simulink model "graduteWork"  (R2019b)
settings: Solver=VariableStepAuto  StartTime=0.0  StopTime=30  RelTol=1e-6  AbsTol=1e-6
values from neighbouring files (symbols this model uses):
  G_0 = db2mag(94)    [apll_attr.m]    (also in apll_const.m = db2mag(90.8); test.m = db2mag(87.3))
  K = 3    [constants.m]    (also in main.m; test.m)
  omega_0 = 0    [apll_attr.m]    (also in apll_const.m; test.m)
  T_b = 2    [constants.m]    (also in main.m)
  tau_p1 = 1.65*1e-3    (= 0.00165)    [apll_attr.m]    (also in apll_attr_nondim_1.m; apll_attr_nondim_2.m; apll_attr_nondim_3.m; apll_const.m)
  tau_p2 = 1.65*1e-3    (= 0.00165)    [apll_attr.m]    (also in apll_attr_nondim_1.m; apll_attr_nondim_2.m; apll_attr_nondim_3.m; apll_const.m)
  tau_z1 = 165*1e-6    (= 0.000165)    [apll_attr.m]    (also in apll_attr_nondim_1.m; apll_attr_nondim_2.m; apll_attr_nondim_3.m; apll_const.m)
  tau_z2 = 165*1e-6    (= 0.000165)    [apll_attr.m]    (also in apll_attr_nondim_1.m; apll_attr_nondim_2.m; apll_attr_nondim_3.m; apll_const.m)
libraries: simulink x3, commrandsrc3 x1, commutil2 x1
settings Model: Creator=Elena  LastModifiedBy=Elena

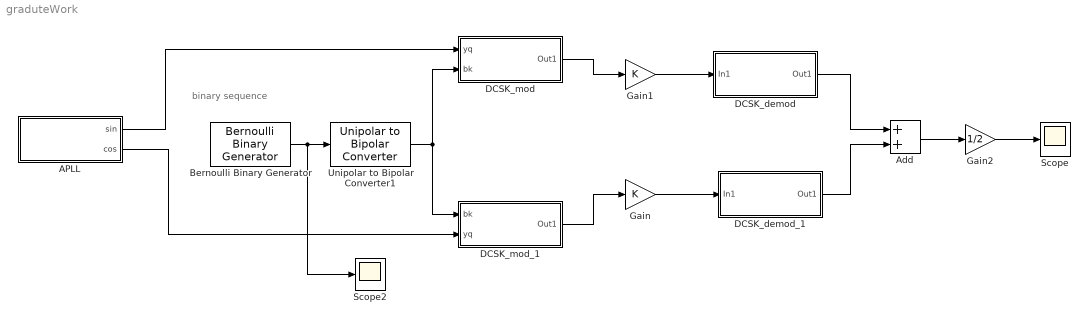
== system graduteWork ==
  note: binary sequence
  "APLL " : Subsystem
  Add : Sum
  Bernoulli Binary Generator : commrandsrc3/Bernoulli Binary Generator  ProbabilityOfZero=0.5  SeedSource=Auto  Seed=0  SampleTime=T_b  SamplesPerFrame=1  OutputDataType=double  SimulateUsing=Interpreted execution
      settings: SourceProductName=Communications Toolbox
  "DCSK_demod " : Subsystem
  "DCSK_demod_1 " : Subsystem
  DCSK_mod : Subsystem
  DCSK_mod_1 : Subsystem
  Gain : Gain  Gain=K
  Gain1 : Gain  Gain=K
  Gain2 : Gain  Gain=1/2
  Scope : Scope
  Scope2 : Scope
  Unipolar to Bipolar Converter1 : commutil2/Unipolar to Bipolar Converter  M=2  polarity=Positive  dataType=Inherit via internal rule
      settings: SourceProductName=Communications Toolbox
  wires:
  "APLL "/1(sin) -> DCSK_mod/1(yq)
  DCSK_mod/1(Out1) -> Gain1/1
  DCSK_mod_1/1(Out1) -> Gain/1
  Add/1 -> Gain2/1
  Unipolar to Bipolar Converter1/1 -> DCSK_mod/2(bk), DCSK_mod_1/1(bk)
  Bernoulli Binary Generator/1 -> Unipolar to Bipolar Converter1/1, Scope2/1
  "APLL "/2(cos) -> DCSK_mod_1/2(yq)
  "DCSK_demod_1 "/1(Out1) -> Add/2
  "DCSK_demod "/1(Out1) -> Add/1
  Gain1/1 -> "DCSK_demod "/1(In1)
  Gain/1 -> "DCSK_demod_1 "/1(In1)
  Gain2/1 -> Scope/1

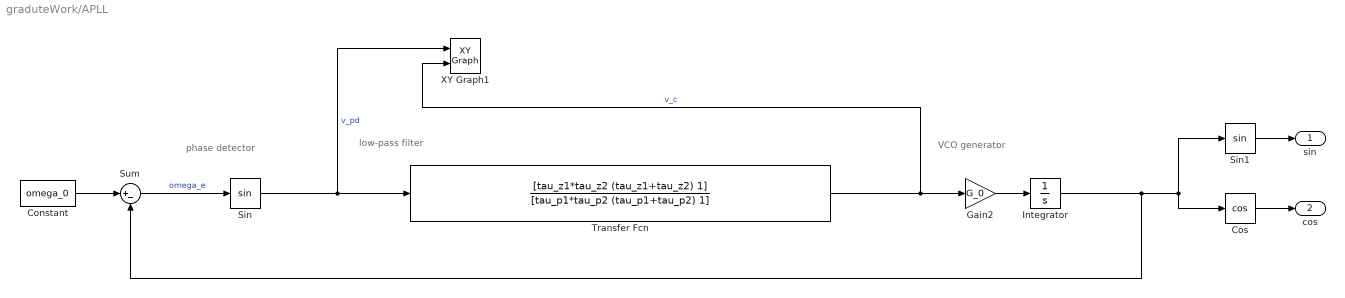
== system graduteWork/APLL  ==
  note: low-pass filter
  note: phase detector
  note: VCO generator
  Constant : Constant  Value=omega_0
  Cos : Trigonometry  Operator=cos
  Gain2 : Gain  Gain=G_0
  Integrator : Integrator  InitialCondition=pi/2
  Sin : Trigonometry
  Sin1 : Trigonometry
  Sum : Sum  Inputs=|+-
  Transfer Fcn : TransferFcn  Numerator=[tau_z1*tau_z2 (tau_z1+tau_z2) 1]  Denominator=[tau_p1*tau_p2 (tau_p1+tau_p2) 1]
  XY Graph1 : simulink/Sinks/XY Graph  xmin=-1  xmax=1  ymin=-1  ymax=1  st=-1
  sin : Outport
  cos : Outport  Port=2
  wires:
  Gain2/1 -> Integrator/1
  Sin/1 -> XY Graph1/1, Transfer Fcn/1  "v_pd"
  Constant/1 -> Sum/1
  Integrator/1 -> Sin1/1, Cos/1, Sum/2
  Transfer Fcn/1 -> XY Graph1/2, Gain2/1  "v_c"
  Sin1/1 -> sin/1
  Sum/1 -> Sin/1  "omega_e"
  Cos/1 -> cos/1

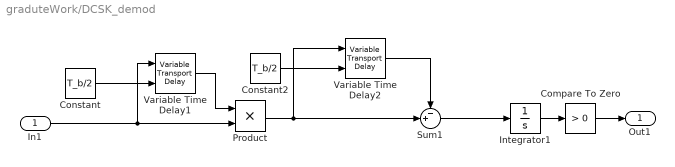
== system graduteWork/DCSK_demod  ==
  In1 : Inport
  Compare To Zero : simulink/Logic and Bit Operations/Compare To Zero  relop=>  OutDataTypeStr=boolean
  Constant : Constant  Value=T_b/2
  Constant2 : Constant  Value=T_b/2
  Integrator1 : Integrator
  Product : Product
  Sum1 : Sum  Inputs=-+|
  Variable Time Delay1 : VariableTransportDelay  MaximumDelay=100
  Variable Time Delay2 : VariableTransportDelay  MaximumDelay=100
  Out1 : Outport
  wires:
  In1/1 -> Product/2, Variable Time Delay1/1
  Variable Time Delay1/1 -> Product/1
  Constant/1 -> Variable Time Delay1/2
  Compare To Zero/1 -> Out1/1
  Constant2/1 -> Variable Time Delay2/2
  Product/1 -> Variable Time Delay2/1, Sum1/2
  Integrator1/1 -> Compare To Zero/1
  Variable Time Delay2/1 -> Sum1/1
  Sum1/1 -> Integrator1/1

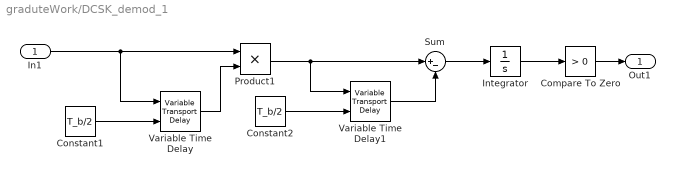
== system graduteWork/DCSK_demod_1  ==
  In1 : Inport
  Compare To Zero : simulink/Logic and Bit Operations/Compare To Zero  relop=>  OutDataTypeStr=boolean
  Constant1 : Constant  Value=T_b/2
  Constant2 : Constant  Value=T_b/2
  Integrator : Integrator
  Product1 : Product
  Sum : Sum  Inputs=|+-
  Variable Time Delay : VariableTransportDelay  MaximumDelay=100
  Variable Time Delay1 : VariableTransportDelay  MaximumDelay=100
  Out1 : Outport
  wires:
  Variable Time Delay/1 -> Product1/2
  Constant1/1 -> Variable Time Delay/2
  In1/1 -> Product1/1, Variable Time Delay/1
  Product1/1 -> Variable Time Delay1/1, Sum/1
  Variable Time Delay1/1 -> Sum/2
  Constant2/1 -> Variable Time Delay1/2
  Sum/1 -> Integrator/1
  Integrator/1 -> Compare To Zero/1
  Compare To Zero/1 -> Out1/1

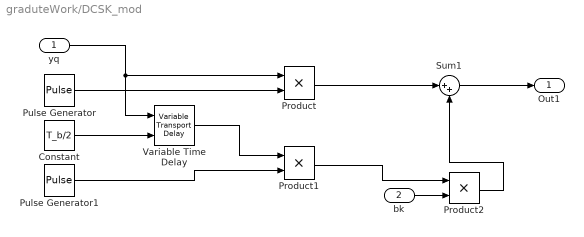
== system graduteWork/DCSK_mod ==
  yq : Inport
  bk : Inport  Port=2
  Constant : Constant  Value=T_b/2
  Product : Product
  Product1 : Product
  Product2 : Product
  Pulse Generator : DiscretePulseGenerator  PulseType=Time based  Period=T_b  PulseWidth=50
  Pulse Generator1 : DiscretePulseGenerator  PulseType=Time based  Period=T_b  PulseWidth=50  PhaseDelay=T_b/2
  Sum1 : Sum  Inputs=|++
  Variable Time Delay : VariableTransportDelay  MaximumDelay=1000
  Out1 : Outport
  wires:
  Sum1/1 -> Out1/1
  yq/1 -> Variable Time Delay/1, Product/1
  Constant/1 -> Variable Time Delay/2
  bk/1 -> Product2/2
  Pulse Generator/1 -> Product/2
  Pulse Generator1/1 -> Product1/2
  Product/1 -> Sum1/1
  Variable Time Delay/1 -> Product1/1
  Product2/1 -> Sum1/2
  Product1/1 -> Product2/1

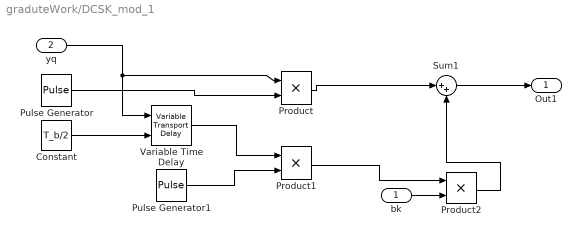
== system graduteWork/DCSK_mod_1 ==
  bk : Inport
  yq : Inport  Port=2
  Constant : Constant  Value=T_b/2
  Product : Product
  Product1 : Product
  Product2 : Product
  Pulse Generator : DiscretePulseGenerator  PulseType=Time based  Period=T_b  PulseWidth=50
  Pulse Generator1 : DiscretePulseGenerator  PulseType=Time based  Period=T_b  PulseWidth=50  PhaseDelay=T_b/2
  Sum1 : Sum  Inputs=|++
  Variable Time Delay : VariableTransportDelay  MaximumDelay=1000
  Out1 : Outport
  wires:
  Constant/1 -> Variable Time Delay/2
  Variable Time Delay/1 -> Product1/1
  Product1/1 -> Product2/1
  Product/1 -> Sum1/1
  Product2/1 -> Sum1/2
  Sum1/1 -> Out1/1
  yq/1 -> Variable Time Delay/1, Product/1
  Pulse Generator/1 -> Product/2
  Pulse Generator1/1 -> Product1/2
  bk/1 -> Product2/2
